simulink model "ValPol5G"  (Simulink 7.0)
settings: Solver=ode3  StartTime=0.0  StopTime=20  FixedStep=0.001  RelTol=1e-3
undefined symbols (not defined in the file or in its folder): CinDirPendulo, CinInvPendulo, JacoboPendulo, pol5G, ScalePol5G, Secuencia4p
settings Model: Creator=dean  LastModifiedBy=dean  ExtModeAutoUpdateStatusClock=off

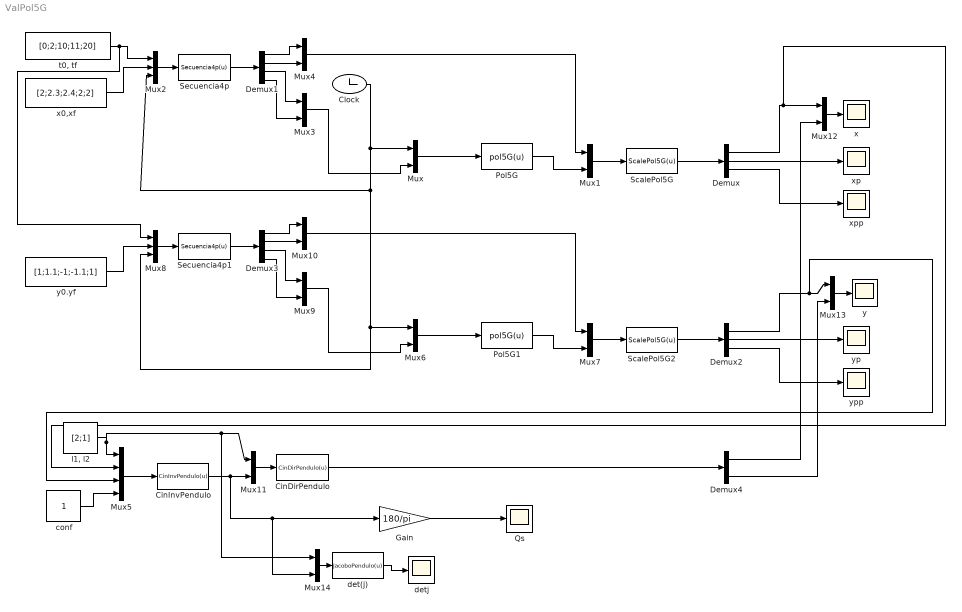
== system ValPol5G ==
  CinDirPendulo : MATLABFcn  MATLABFcn=CinDirPendulo(u)  OutputDimensions=2
  CinInvPendulo : MATLABFcn  MATLABFcn=CinInvPendulo(u)  OutputDimensions=2
  Clock : Clock
      settings: Decimation=10
  Demux : Demux  Outputs=3
  Demux1 : Demux
  Demux2 : Demux  Outputs=3
  Demux3 : Demux
  Demux4 : Demux  Outputs=2
  Gain : Gain  Gain=180/pi  ParameterDataType=sfix(16)  ParameterScaling=2^0  OutDataType=sfix(16)  OutScaling=2^0
  Mux{,1,3..4,6..7,9..14} (12 alike) : Mux  Inputs=2
  Mux2 : Mux  Inputs=3
  Mux5 : Mux
  Mux8 : Mux  Inputs=3
  Pol5G : MATLABFcn  MATLABFcn=pol5G(u)  OutputDimensions=3
  Pol5G1 : MATLABFcn  MATLABFcn=pol5G(u)  OutputDimensions=3
  Qs : Scope
      settings: TimeRange=20  YMax=105  SaveName=ScopeData6
  ScalePol5G : MATLABFcn  MATLABFcn=ScalePol5G(u)  OutputDimensions=3
  ScalePol5G2 : MATLABFcn  MATLABFcn=ScalePol5G(u)  OutputDimensions=3
  Secuencia4p : MATLABFcn  MATLABFcn=Secuencia4p(u)  OutputDimensions=4
  Secuencia4p1 : MATLABFcn  MATLABFcn=Secuencia4p(u)  OutputDimensions=4
  conf : Constant  OutDataType=sfix(16)  OutScaling=2^0
  det(j) : MATLABFcn  MATLABFcn=JacoboPendulo(u)  OutputDimensions=1
  detj : Scope
      settings: TimeRange=20  YMax=105  SaveName=ScopeData7
  "l1, l2" : Constant  Value=[2;1]  OutDataType=sfix(16)  OutScaling=2^0
  "t0, tf" : Constant  Value=[0;2;10;11;20]  OutDataType=sfix(16)  OutScaling=2^0
  x : Scope
      settings: TimeRange=20  YMin=1.975  YMax=2.425
  x0,xf : Constant  Value=[2;2.3;2.4;2;2]  OutDataType=sfix(16)  OutScaling=2^0
  xp : Scope
  xpp : Scope
      settings: SaveName=ScopeData2
  y : Scope
      settings: TimeRange=20  YMin=-1.25  YMax=1.25  SaveName=ScopeData3
  y0.yf : Constant  Value=[1;1.1;-1;-1.1;1]  OutDataType=sfix(16)  OutScaling=2^0
  yp : Scope
      settings: SaveName=ScopeData4
  ypp : Scope
      settings: SaveName=ScopeData5
  wires:
  Mux/1 -> Pol5G/1
  Demux/1 -> Mux12/1, Mux5/2
  Demux/2 -> xp/1
  Demux/3 -> xpp/1
  Clock/1 -> Mux/1, Mux2/3, Mux6/1, Mux8/3
  Mux1/1 -> ScalePol5G/1
  Pol5G/1 -> Mux1/2
  ScalePol5G/1 -> Demux/1
  Mux2/1 -> Secuencia4p/1
  "t0, tf"/1 -> Mux2/1, Mux8/1
  x0,xf/1 -> Mux2/2
  Secuencia4p/1 -> Demux1/1
  Demux1/1 -> Mux4/1
  Demux1/2 -> Mux4/2
  Demux1/3 -> Mux3/1
  Demux1/4 -> Mux3/2
  Mux3/1 -> Mux/2
  Mux4/1 -> Mux1/1
  Mux5/1 -> CinInvPendulo/1
  Mux6/1 -> Pol5G1/1
  Demux2/1 -> Mux13/1, Mux5/3
  Demux2/2 -> yp/1
  Demux2/3 -> ypp/1
  Mux7/1 -> ScalePol5G2/1
  Pol5G1/1 -> Mux7/2
  ScalePol5G2/1 -> Demux2/1
  Mux8/1 -> Secuencia4p1/1
  y0.yf/1 -> Mux8/2
  Secuencia4p1/1 -> Demux3/1
  Demux3/1 -> Mux10/1
  Demux3/2 -> Mux10/2
  Demux3/3 -> Mux9/1
  Demux3/4 -> Mux9/2
  Mux9/1 -> Mux6/2
  Mux10/1 -> Mux7/1
  "l1, l2"/1 -> Mux5/1, Mux11/1, Mux14/1
  Mux11/1 -> CinDirPendulo/1
  CinInvPendulo/1 -> Mux11/2, Gain/1, Mux14/2
  CinDirPendulo/1 -> Demux4/1
  Mux12/1 -> x/1
  Demux4/1 -> Mux12/2
  Mux13/1 -> y/1
  Demux4/2 -> Mux13/2
  conf/1 -> Mux5/4
  Gain/1 -> Qs/1
  Mux14/1 -> det(j)/1
  det(j)/1 -> detj/1
